simulink model "Exercitiul1"  (R2016a)
settings: Solver=VariableStepDiscrete  StartTime=0.0  StopTime=240  RelTol=1e-3
undefined symbols (not defined in the file): m, n
settings Model: Creator=Cristina  LastModifiedBy=Cristina

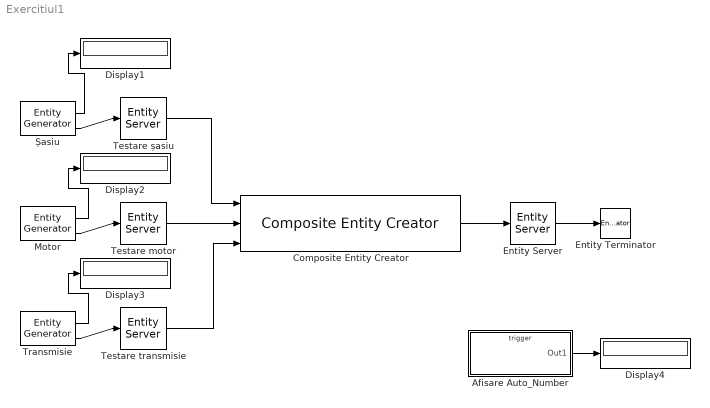
== system Exercitiul1 ==
  Afisare Auto_Number : Subsystem  TreatAsAtomicUnit=on
  Composite Entity Creator : CompositeEntityCreator  InputPortMessageModes=m,m,m  OutputPortMessageModes=m  NumberInputPorts=3  EntityTypeName=Combined  InputEntityName=Sasiu|Motor|Transmisie
      settings: InputPortMap=u0,u1,u2
  Display{1..4} (4 alike) : Display
  Entity Server : EntityServer  InputPortMessageModes=m  OutputPortMessageModes=m  Capacity=1  ServiceTimeValue=0.3  ServiceCompleteAction=|
      | entity.Sasiu.Auto_Number = ...
      |     entity.Motor.Motor_Nbr + ...
      |     (entity.Transmisie.Transmisie_Nbr) * 10 + ...
      |     (entity.Sasiu.Sasiu_Nbr) + 100;
      | f(entity.Sasiu.Auto_Number);
  Entity Terminator : EntityTerminator  InputPortMessageModes=m
  Motor : EntityGenerator  OutputPortMessageModes=n,m  Period=0.8  GenerateAction=|  AttributeName=Motor_Nbr  NumberEntitiesDeparted=on  EntityType=Structured  EntityTypeName=Motor
      | persistent Motor_count
      | if (isempty(Motor_count))
      |     Motor_count = 0;
      | end
      | Motor_count = Motor_count + 1;
      | entity.Motor_Nbr = Motor_count;
      settings: OutputPortMap=o0,o3
  Testare motor : EntityServer  InputPortMessageModes=m  OutputPortMessageModes=m  Capacity=1  ServiceTimeValue=0.6
  Testare transmisie : EntityServer  InputPortMessageModes=m  OutputPortMessageModes=m  Capacity=1  ServiceTimeValue=0.4
  Testare șasiu : EntityServer  InputPortMessageModes=m  OutputPortMessageModes=m  Capacity=1  ServiceTimeValue=0.4
  Transmisie : EntityGenerator  OutputPortMessageModes=n,m  Period=0.6  GenerateAction=|  AttributeName=Transmisie_Nbr  NumberEntitiesDeparted=on  EntityType=Structured  EntityTypeName=Transmisie
      | persistent Transmisie_count
      | if (isempty(Transmisie_count))
      |     Transmisie_count = 0;
      | end
      | Transmisie_count = Transmisie_count + 1;
      | entity.Transmisie_Nbr = Transmisie_count;
      settings: OutputPortMap=o0,o3
  Șasiu : EntityGenerator  OutputPortMessageModes=n,m  Period=0.4  GenerateAction=|  AttributeName=Sasiu_Nbr|Auto_Number  AttributeInitialValue=1|0  NumberEntitiesDeparted=on  EntityType=Structured  EntityTypeName=Sasiu
      | persistent Sasiu_count
      | if (isempty(Sasiu_count))
      |     Sasiu_count = 0;
      | end
      | Sasiu_count = Sasiu_count + 1;
      | entity.Sasiu_Nbr = Sasiu_count;
      settings: OutputPortMap=o0,o3
  wires:
  Șasiu/2 -> Testare șasiu/1
  Motor/2 -> Testare motor/1
  Transmisie/2 -> Testare transmisie/1
  Composite Entity Creator/1 -> Entity Server/1
  Entity Server/1 -> Entity Terminator/1
  Testare șasiu/1 -> Composite Entity Creator/1
  Testare motor/1 -> Composite Entity Creator/2
  Testare transmisie/1 -> Composite Entity Creator/3
  Șasiu/1 -> Display1/1
  Motor/1 -> Display2/1
  Transmisie/1 -> Display3/1
  Afisare Auto_Number/1(Out1) -> Display4/1

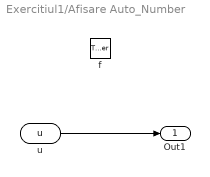
== system Exercitiul1/Afisare Auto_Number ==
  f : TriggerPort  TriggerType=function-call  IsSimulinkFunction=on  FunctionName=f  VariantControl=Variant
  u : ArgIn  DisableCoverage=on  ArgumentName=u
  Out1 : Outport
  wires:
  u/1 -> Out1/1
